simulink model "Template"  (R2023a)
settings: Solver=VariableStepAuto  StartTime=0.0  StopTime=3*Ts  FixedStep=dt  MaxStep=dt  RelTol=1e-5  EnableMultiTasking=on
values from neighbouring files (symbols this model uses):
  Ar = A    [Skelaton.m]
  B = [0;1]    [Skelaton.m]
  Bss = (B'*B)^-1*B'*A    [Skelaton.m]
  C = [1 0]    [Skelaton.m]
  dt = 0.01    [Skelaton.m]
  K = place(A,B,poles_b)    [Skelaton.m]
  Kd = place(Ad,Bd,Pd)    [Skelaton.m]
settings Model: Creator=Andrew Petruska  LastModifiedBy=Tanmay
settings SolverCC: AlgebraicLoopSolver=TrustRegion
settings DataIOCC: ReturnWorkspaceOutputs=off
settings OptimizationCC: LifeSpan=inf
settings DebuggingCC: UnconnectedInputMsg=warning  UnconnectedOutputMsg=warning  UnconnectedLineMsg=warning  SFUnexpectedBacktrackingDiag=warning  SFNoUnconditionalDefaultTransitionDiag=warning  ArithmeticOperatorsInVariantConditions=warning
settings ModelReferenceCC: EnableRefExpFcnMdlSchedulingChecks=on
settings SFSimCC: SimUseLocalCustomCode=off  CustomCodeUndefinedFunction=UseInterfaceOnly
settings RTWCC: RTWUseLocalCustomCode=off
settings CodeAppCC: StateflowObjectComments=on
settings GRTTargetCC: TargetLangStandard=C89/C90 (ANSI)
settings ConfigComp: CovMetricSettings=dw  CovSaveCumulativeToWorkspaceVar=on  CovSaveSingleToWorkspaceVar=on  CovExternalEMLEnable=off

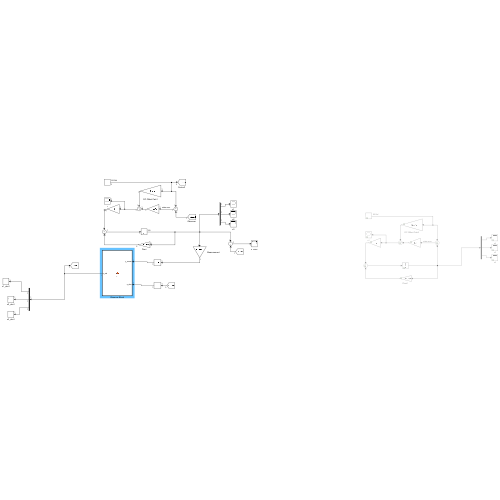
[thumbnail: Simulink's stored preview of the top-level diagram]
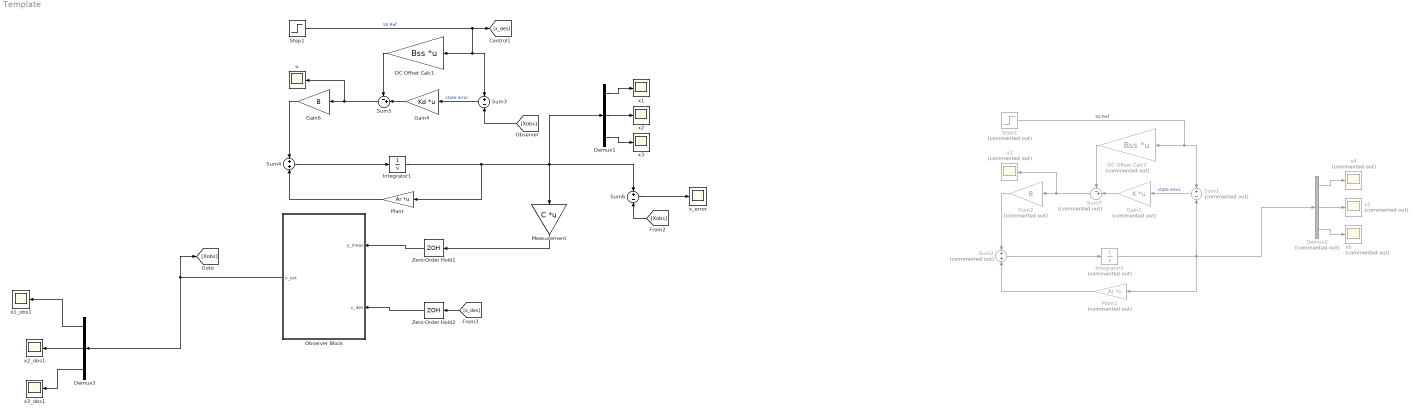
== system Template ==
  DC Offset Calc1 : Gain  Gain=Bss  Multiplication=Matrix(K*u)
  DC Offset Calc2 : Gain  Commented=on  Gain=Bss  Multiplication=Matrix(K*u)
  Demux1 : Demux  Outputs=3
  Demux2 : Demux  Commented=on  Outputs=3
  Demux3 : Demux  Outputs=3
  Gain1 : Gain  Commented=on  Gain=K  Multiplication=Matrix(K*u)
  Gain2 : Gain  Commented=on  Gain=B
  Gain4 : Gain  Gain=Kd  Multiplication=Matrix(K*u)
  Gain6 : Gain  Gain=B
  Integrator1 : Integrator  InitialCondition=[0;0;0]
  Integrator2 : Integrator  Commented=on  InitialCondition=[0;0]
  Measurement : Gain  Gain=C  Multiplication=Matrix(K*u) (u vector)
  "Observer Block " : MATLAB Function  TreatAsAtomicUnit=on
  Plant : Gain  Gain=Ar  Multiplication=Matrix(K*u) (u vector)
  Plant1 : Gain  Commented=on  Gain=Ar  Multiplication=Matrix(K*u) (u vector)
  Step1 : Step  Time=0  After=[1;0;0]  SampleTime=dt
  Step2 : Step  Commented=on  Time=[1;0]  SampleTime=0
  Sum1 : Sum  Commented=on  Inputs=+-
  Sum2 : Sum  Commented=on  Inputs=+|+
  Sum3 : Sum  Inputs=+-
  Sum4 : Sum  Inputs=+|+
  Sum5 : Sum  Inputs=-+|
  Sum6 : Sum  Inputs=+-
  Sum7 : Sum  Commented=on  Inputs=-+|
  Zero-Order Hold1 : ZeroOrderHold  SampleTime=dt
  Zero-Order Hold2 : ZeroOrderHold  SampleTime=dt
  u : Scope
  u1 : Scope  Commented=on
  x1 : Scope
  x1_obs1 : Scope
  x2 : Scope
  x2_obs1 : Scope
  x3 : Scope
  x3_obs1 : Scope
  x4 : Scope  Commented=on
  x5 : Scope  Commented=on
  x6 : Scope  Commented=on
  x_error : Scope
  wires:
  Step1/1 -> Sum3/1, DC Offset Calc1/1, [x_des]  "SS Ref"
  Plant/1 -> Sum4/2
  Sum4/1 -> Integrator1/1
  Integrator1/1 -> Plant/1, Measurement/1, Sum6/1, Demux1/1
  Demux1/1 -> x1/1
  Demux1/2 -> x2/1
  Demux1/3 -> x3/1
  Sum3/1 -> Gain4/1  "state error"
  Gain6/1 -> Sum4/1
  Gain4/1 -> Sum5/2
  DC Offset Calc1/1 -> Sum5/1
  Sum5/1 -> u/1, Gain6/1
  Measurement/1 -> Zero-Order Hold1/1
  Zero-Order Hold1/1 -> "Observer Block "/1(y_meas)
  [Xobs] -> Sum3/2
  Sum6/1 -> x_error/1
  [Xobs] -> Sum6/2
  Demux3/2 -> x2_obs1/1
  Demux3/3 -> x3_obs1/1
  Demux3/1 -> x1_obs1/1
  "Observer Block "/1(x_est) -> Demux3/1, [Xobs]
  [x_des] -> Zero-Order Hold2/1
  Zero-Order Hold2/1 -> "Observer Block "/2(x_des)
  DC Offset Calc2/1 -> Sum7/1
  Demux2/2 -> x5/1
  Step2/1 -> Sum1/1, DC Offset Calc2/1  "SS Ref"
  Gain1/1 -> Sum7/2
  Sum7/1 -> u1/1, Gain2/1
  Plant1/1 -> Sum2/2
  Demux2/3 -> x6/1
  Gain2/1 -> Sum2/1
  Integrator2/1 -> Sum1/2, Demux2/1, Plant1/1
  Sum2/1 -> Integrator2/1
  Demux2/1 -> x4/1
  Sum1/1 -> Gain1/1  "state error"

== matlab function Template/Observer Block  ==
  data: y_meas input; x_est output; x_des input
function x_est  = fcn(y_meas, x_des)
%#codegen,
coder.extrinsic('evalin');
persistent Ad Bd C L Kd Bss x_last;% Ki int_sat x_sum;

if isempty(Ad) || isempty(Bd) || isempty(C) || isempty(L) ||isempty(x_last) %|| isempty(x_sum)
    % Initialize Size of System from Workspace
    Ad = zeros(3,3);
    Bd = zeros(3,1);
    C  = zeros(1,3);
    L  = zeros(3,1);
    Kd = zeros(1,3);
    Bss = zeros(1,3);
%     Ki  = 0;
%     int_sat = 0; % for integrator
    
    % Read Values from Workspace
    Ad = evalin('base','Ad');
    Bd = evalin('base','Bd');
    C = evalin('base','C');
    L = evalin('base','L');
    Kd = evalin('base','Kd');
    Bss = evalin('base','Bss');
%     Ki = evalin('base','Ki');
%     int_sat = evalin('base','int_sat');
    
    % initialize observer to Zeros
    x_last = zeros(3,1);
%     x_sum = zeros(1,1); % for intergrator 
    
    x_est = x_last;% initial output is zero
%     x_int = x_sum; %initial ouput is zero

    
else
    
    % Calculate Control that was applied
    u_k = Kd*(x_des-x_last)-Bss*x_des;
%     u_k = u_k + Ki*x_sum; %add in integrator
    
    % Calculate model update
    x_est = Ad*x_last + Bd*u_k; % model update
    x_est = x_est + L*(y_meas - C*x_est); % measurement update
    
    % Put model update out to the world
    x_last = x_est;
    
%     % For an Integrator
%     x_sum = x_sum + C*(x_des-x_est);
%     
%     % Prevent Windup
%     if x_sum > int_sat
%         x_sum = int_sat;
%     elseif x_sum < -int_sat
%         x_sum = -int_sat;
%     end
%     
%     % return integration
%      x_int = x_sum;
    
end
